simulink model "fft_ins_outs"  (Simulink 5.0)
settings: Solver=FixedStepDiscrete  StartTime=0.0  StopTime=1  RelTol=1e-3
libraries: dspsrcs4 x4, dspxfrm3 x4
settings Model: CovMetricSettings=d  Creator=ckamachi  LastModifiedBy=ckamachi  BooleanDataType=off

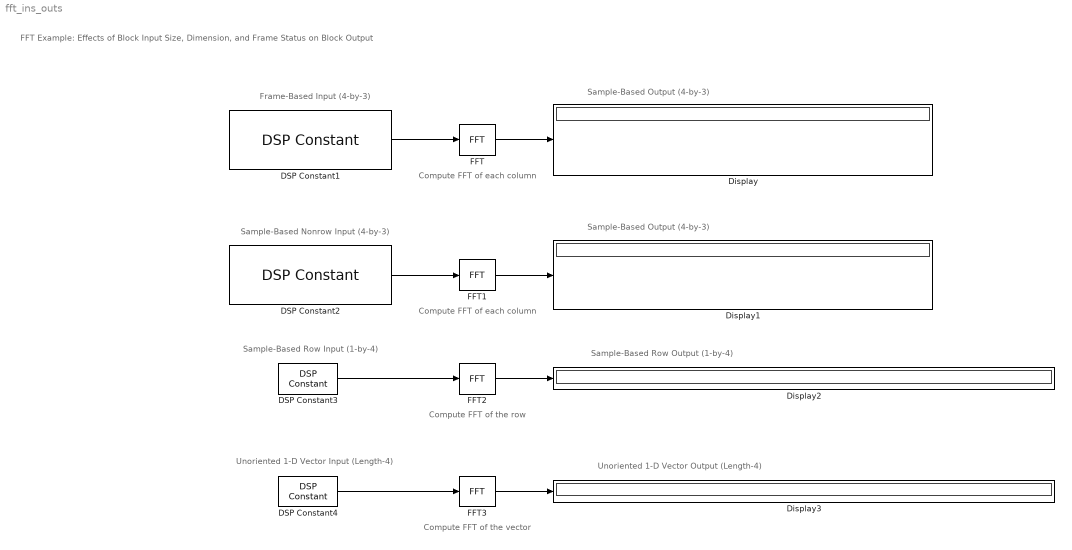
== system fft_ins_outs ==
  note: Frame-Based Input (4-by-3)
  note: Sample-Based Nonrow Input (4-by-3)
  note: Sample-Based Row Input (1-by-4)
  note: Unoriented 1-D Vector Input (Length-4)
  note: Sample-Based Output (4-by-3)
  note: Sample-Based Output (4-by-3)
  note: Sample-Based Row Output (1-by-4)
  note: Unoriented 1-D Vector Output (Length-4)
  note: FFT Example:
      | Effects of Block Input Size, Dimension, and Frame Status on Block Output
  note: Compute FFT of each column
  note: Compute FFT of each column
  note: Compute FFT of the row
  note: Compute FFT of the vector
  DSP Constant1 : dspsrcs4/DSP Constant  Value=[1 2 3 4; 2 4 6 8; 3 6 9 12]'  SampleMode=Discrete  discreteOutput=Frame-based  continuousOutput=Sample-based  sampTime=1  framePeriod=1  dataType=Inherit from 'Constant value'  wordLen=16  udDataType=sfix(16)  fracBitsMode=Best precision  numFracBits=15  InterpretAs1D=off  Ts=1  FramebasedOutput=on
  DSP Constant2 : dspsrcs4/DSP Constant  Value=[1 2 3 4; 2 4 6 8; 3 6 9 12]'  SampleMode=Discrete  discreteOutput=Sample-based  continuousOutput=Sample-based  sampTime=1  framePeriod=1  dataType=Inherit from 'Constant value'  wordLen=16  udDataType=sfix(16)  fracBitsMode=Best precision  numFracBits=15  InterpretAs1D=off  Ts=1  FramebasedOutput=off
  DSP Constant3 : dspsrcs4/DSP Constant  Value=[1 2 3 4]  SampleMode=Discrete  discreteOutput=Sample-based  continuousOutput=Sample-based  sampTime=1  framePeriod=1  dataType=Inherit from 'Constant value'  wordLen=16  udDataType=sfix(16)  fracBitsMode=Best precision  numFracBits=15  InterpretAs1D=off  Ts=1  FramebasedOutput=off
  DSP Constant4 : dspsrcs4/DSP Constant  Value=[1 2 3 4]  SampleMode=Discrete  discreteOutput=Sample-based (interpret vectors as 1-D)  continuousOutput=Sample-based (interpret vectors as 1-D)  sampTime=1  framePeriod=1  dataType=Inherit from 'Constant value'  wordLen=16  udDataType=sfix(16)  fracBitsMode=Best precision  numFracBits=15  InterpretAs1D=on  Ts=1  FramebasedOutput=off
  Display{,1..3} (4 alike) : Display
  FFT{,1..3} (4 alike) : dspxfrm3/FFT  CompMethod=Table lookup  TableOpt=Speed  BitRevOrder=off
  wires:
  DSP Constant1/1 -> FFT/1
  FFT/1 -> Display/1
  DSP Constant2/1 -> FFT1/1
  FFT1/1 -> Display1/1
  DSP Constant3/1 -> FFT2/1
  FFT2/1 -> Display2/1
  DSP Constant4/1 -> FFT3/1
  FFT3/1 -> Display3/1
